simulink model "LunarLanderLQRKalman"  (R2022b)
settings: Solver=ode45  StartTime=0.0  StopTime=50  RelTol=1e-2
undefined symbols (not defined in the file): A, B, C, Kp, L, L_tK
libraries: simulink x4
settings Model: Creator=marco  LastModifiedBy=marco

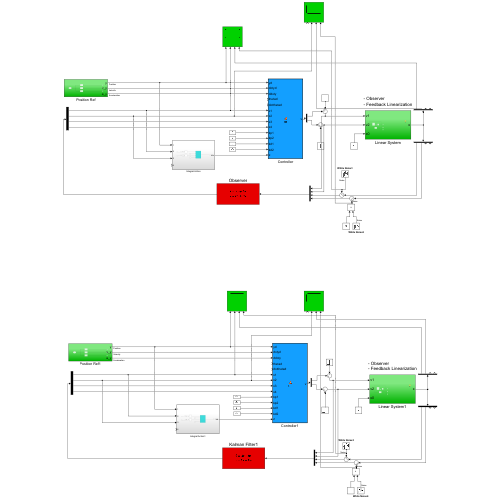
[thumbnail: Simulink's stored preview of the top-level diagram]
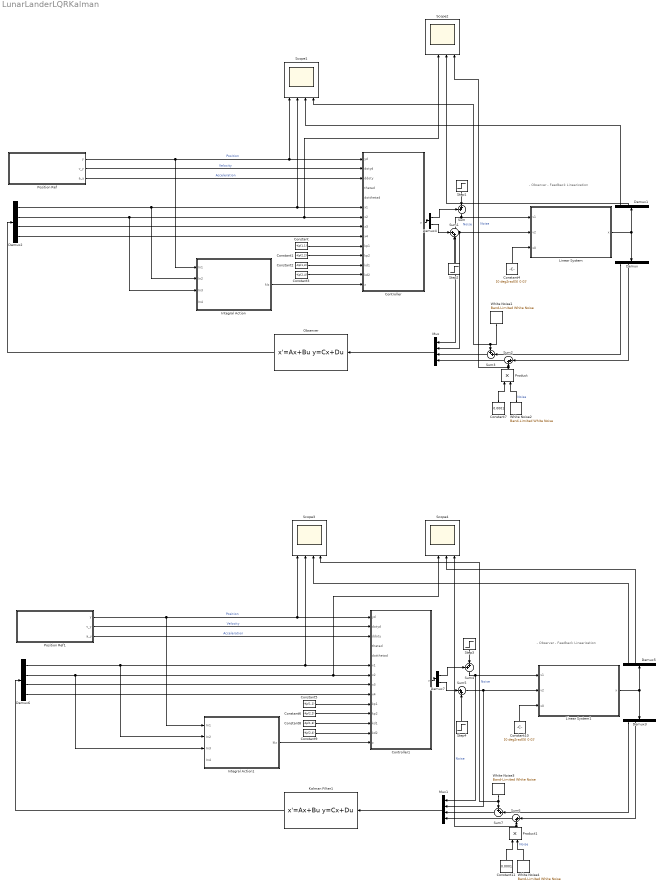
== system LunarLanderLQRKalman ==
  note: - Observer
      | - Feedback Linearization
  note: - Observer
      | - Feedback Linearization
  Constant : Constant  Value=-Kp(1,1)
  Constant1 : Constant  Value=-Kp(2,2)
  Constant10 : Constant  Value=[0 deg2rad(5) 0 0]'
  Constant11 : Constant  Value=0.0001
  Constant2 : Constant  Value=-Kp(1,3)
  Constant3 : Constant  Value=-Kp(2,4)
  Constant4 : Constant  Value=[0 deg2rad(5) 0 0]'
  Constant5 : Constant  Value=-Kp(1,1)
  Constant6 : Constant  Value=-Kp(2,2)
  Constant7 : Constant  Value=0.0001
  Constant8 : Constant  Value=-Kp(1,3)
  Constant9 : Constant  Value=-Kp(2,4)
  Controller : MATLAB Function  TreatAsAtomicUnit=on
  Controller1 : MATLAB Function  TreatAsAtomicUnit=on
  Demux{,1..3,5..6} (6 alike) : Demux
  Demux4 : Demux  Outputs=2
  Demux7 : Demux  Outputs=2
  Integral Action : Subsystem
  Integral Action1 : Subsystem
  Kalman Filter1 : StateSpace  A=A-L_tK*C  B=[B L_tK]  C=eye(4)  D=zeros(4)  InitialCondition=0
  Linear System : Subsystem
  Linear System1 : Subsystem
  Mux : Mux
  Mux1 : Mux
  Observer : StateSpace  A=A-L*C  B=[B L]  C=eye(4)  D=zeros(4)  InitialCondition=0
  Position Ref : Subsystem
  Position Ref1 : Subsystem
  Product : Product
  Product1 : Product
  Scope{1..4} (4 alike) : Scope  NumInputPorts=4
  Step1 : Step  After=10  SampleTime=0
  Step2 : Step  After=deg2rad(1)  SampleTime=0
  Step3 : Step  After=10  SampleTime=0
  Step4 : Step  After=deg2rad(1)  SampleTime=0
  Sum{,3..4,7} (4 alike) : Sum  Inputs=++|
  Sum{1..2,5..6} (4 alike) : Sum  Inputs=|++
  White Noise{1..4} (4 alike) : simulink/Sources/Band-Limited White Noise  Cov=[2]  Ts=0.1  seed=[213132]
  wires:
  Constant7/1 -> Product/1
  White Noise2/1 -> Product/2  "Noise"
  Position Ref/1(y) -> Controller/1(yd), Scope1/1, Integral Action/1(In1)  "Position"
  Demux4/1 -> Sum/1
  Demux1/2 -> Scope2/3
  Mux/1 -> Observer/1
  Sum1/1 -> Linear System/2(v2), Mux/2
  Integral Action/1(kIz) -> Controller/14(z)
  Controller/1(v) -> Demux4/1
  Demux2/4 -> Controller/9(x4)
  Constant1/1 -> Controller/11(kp2)
  Constant2/1 -> Controller/12(kd1)
  Constant4/1 -> Linear System/3(x0)
  Position Ref/3(a_y) -> Controller/3(ddoty)  "Acceleration"
  Observer/1 -> Demux2/1
  Position Ref/2(v_y) -> Controller/2(dotyd)  "Velocity"
  Demux2/3 -> Controller/8(x3)
  Constant3/1 -> Controller/13(kd2)
  Linear System/1(x) -> Demux/1, Demux1/1
  Demux/1 -> Sum3/2
  Demux1/1 -> Scope1/3
  Step1/1 -> Sum/2
  Constant/1 -> Controller/10(kp1)
  Demux4/2 -> Sum1/1
  Demux2/2 -> Controller/7(x2), Scope2/2, Integral Action/3(In3)
  Sum/1 -> Linear System/1(v1), Mux/1
  Demux2/1 -> Scope1/2, Controller/6(x1), Integral Action/2(In2)
  Step2/1 -> Sum1/2
  Demux/2 -> Sum2/1
  Sum2/1 -> Mux/4
  Product/1 -> Scope2/4, Sum2/2  "Noise"
  Sum3/1 -> Mux/3
  White Noise1/1 -> Scope1/4, Sum3/1  "Noise"
  Constant8/1 -> Controller1/12(kd1)
  Integral Action1/1(kIz) -> Controller1/14(z)
  Controller1/1(v) -> Demux7/1
  Sum5/1 -> Mux1/2, Linear System1/2(v2)
  Constant5/1 -> Controller1/10(kp1)
  Demux7/2 -> Sum5/1
  Sum4/1 -> Mux1/1, Linear System1/1(v1)
  Demux6/2 -> Scope4/2, Controller1/7(x2), Integral Action1/3(In3)
  Constant9/1 -> Controller1/13(kd2)
  Position Ref1/2(v_y) -> Controller1/2(dotyd)  "Velocity"
  Kalman Filter1/1 -> Demux6/1
  Step3/1 -> Sum4/2
  Linear System1/1(x) -> Demux3/1, Demux5/1
  Position Ref1/3(a_y) -> Controller1/3(ddoty)  "Acceleration"
  Demux6/3 -> Controller1/8(x3)
  Position Ref1/1(y) -> Controller1/1(yd), Scope3/1, Integral Action1/1(In1)  "Position"
  Sum7/1 -> Mux1/3
  Demux6/4 -> Controller1/9(x4)
  Demux3/2 -> Sum6/1
  Demux5/2 -> Scope4/3
  Step4/1 -> Sum5/2
  Demux7/1 -> Sum4/1
  Demux6/1 -> Scope3/2, Controller1/6(x1), Integral Action1/2(In2)
  Mux1/1 -> Kalman Filter1/1
  Demux3/1 -> Sum7/2
  White Noise4/1 -> Product1/2  "Noise"
  Constant11/1 -> Product1/1
  Sum6/1 -> Mux1/4
  Constant10/1 -> Linear System1/3(x0)
  Product1/1 -> Scope4/4, Sum6/2  "Noise"
  White Noise3/1 -> Scope3/4, Sum7/1  "Noise"
  Constant6/1 -> Controller1/11(kp2)
  Demux5/1 -> Scope3/3

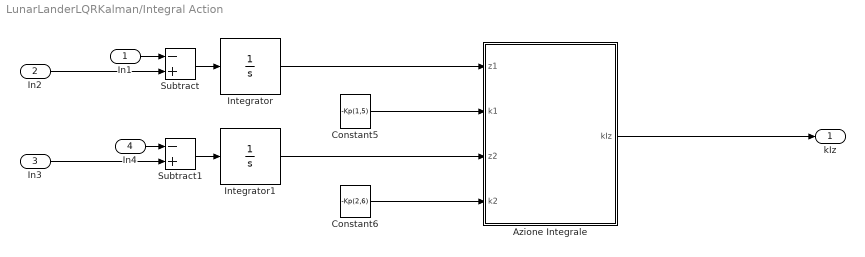
== system LunarLanderLQRKalman/Integral Action ==
  In1 : Inport
  In2 : Inport  Port=2
  In3 : Inport  Port=3
  In4 : Inport  Port=4
  Azione Integrale : MATLAB Function  TreatAsAtomicUnit=on
  Constant5 : Constant  Value=-Kp(1,5)
  Constant6 : Constant  Value=-Kp(2,6)
  Integrator : Integrator
  Integrator1 : Integrator
  Subtract : Sum  Inputs=-+
  Subtract1 : Sum  Inputs=-+
  kIz : Outport
  wires:
  Integrator/1 -> Azione Integrale/1(z1)
  Constant6/1 -> Azione Integrale/4(k2)
  Integrator1/1 -> Azione Integrale/3(z2)
  Subtract1/1 -> Integrator1/1
  Constant5/1 -> Azione Integrale/2(k1)
  Subtract/1 -> Integrator/1
  In3/1 -> Subtract1/2
  In4/1 -> Subtract1/1
  In1/1 -> Subtract/1
  Azione Integrale/1(kIz) -> kIz/1
  In2/1 -> Subtract/2

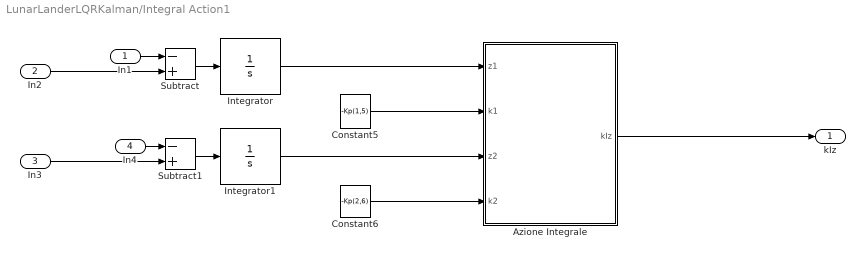
== system LunarLanderLQRKalman/Integral Action1 ==
  In1 : Inport
  In2 : Inport  Port=2
  In3 : Inport  Port=3
  In4 : Inport  Port=4
  Azione Integrale : MATLAB Function  TreatAsAtomicUnit=on
  Constant5 : Constant  Value=-Kp(1,5)
  Constant6 : Constant  Value=-Kp(2,6)
  Integrator : Integrator
  Integrator1 : Integrator
  Subtract : Sum  Inputs=-+
  Subtract1 : Sum  Inputs=-+
  kIz : Outport
  wires:
  Integrator/1 -> Azione Integrale/1(z1)
  Constant6/1 -> Azione Integrale/4(k2)
  Integrator1/1 -> Azione Integrale/3(z2)
  Subtract1/1 -> Integrator1/1
  Constant5/1 -> Azione Integrale/2(k1)
  Subtract/1 -> Integrator/1
  In3/1 -> Subtract1/2
  In4/1 -> Subtract1/1
  In1/1 -> Subtract/1
  Azione Integrale/1(kIz) -> kIz/1
  In2/1 -> Subtract/2

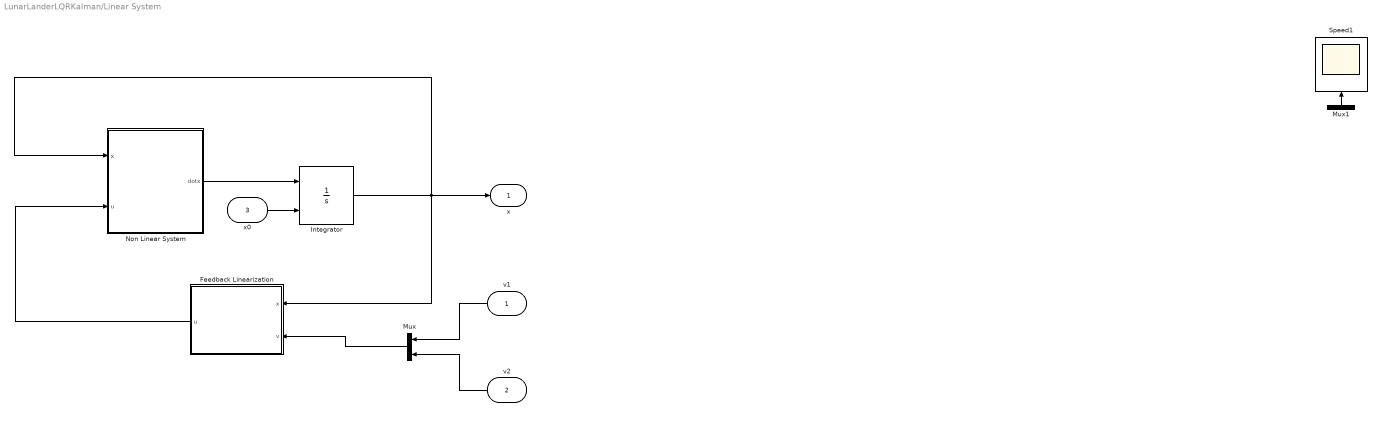
== system LunarLanderLQRKalman/Linear System ==
  v1 : Inport
  v2 : Inport  Port=2
  x0 : Inport  Port=3
  Feedback Linearization : MATLAB Function  TreatAsAtomicUnit=on
  Integrator : Integrator  InitialConditionSource=external  InitialCondition=[0 0 0 0]'
  Mux : Mux  Inputs=2
  Mux1 : Mux  Inputs=2
  Non Linear System : MATLAB Function  TreatAsAtomicUnit=on
  Speed1 : Scope
  x : Outport
  wires:
  Feedback Linearization/1(u) -> Non Linear System/2(u)
  Integrator/1 -> Non Linear System/1(x), x/1, Feedback Linearization/1(x)
  Non Linear System/1(dotx) -> Integrator/1
  x0/1 -> Integrator/2
  v1/1 -> Mux/1
  v2/1 -> Mux/2
  Mux/1 -> Feedback Linearization/2(v)
  Mux1/1 -> Speed1/1

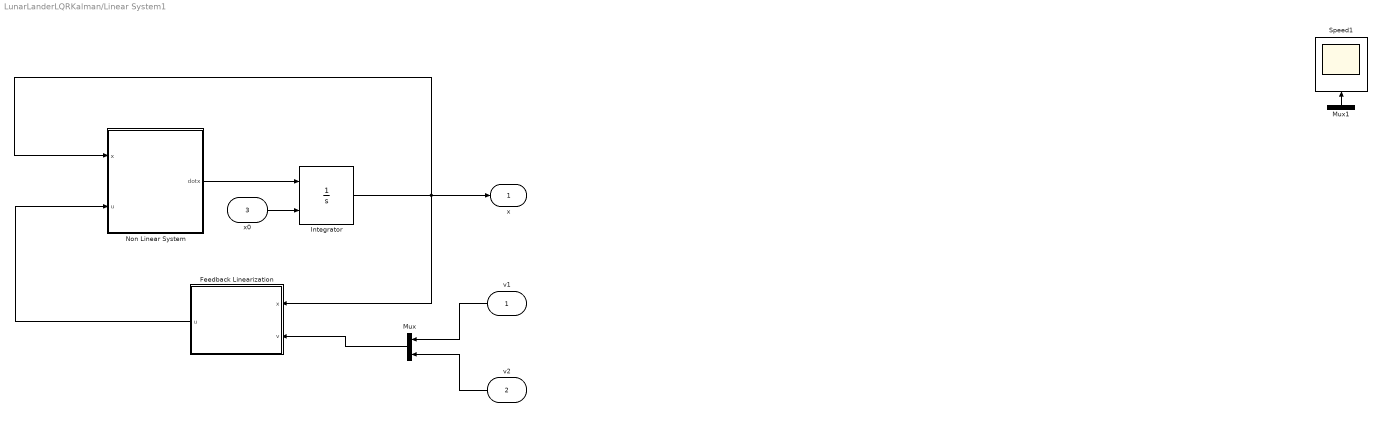
== system LunarLanderLQRKalman/Linear System1 ==
  v1 : Inport
  v2 : Inport  Port=2
  x0 : Inport  Port=3
  Feedback Linearization : MATLAB Function  TreatAsAtomicUnit=on
  Integrator : Integrator  InitialConditionSource=external  InitialCondition=[0 0 0 0]'
  Mux : Mux  Inputs=2
  Mux1 : Mux  Inputs=2
  Non Linear System : MATLAB Function  TreatAsAtomicUnit=on
  Speed1 : Scope
  x : Outport
  wires:
  Feedback Linearization/1(u) -> Non Linear System/2(u)
  Integrator/1 -> Non Linear System/1(x), x/1, Feedback Linearization/1(x)
  Non Linear System/1(dotx) -> Integrator/1
  x0/1 -> Integrator/2
  v1/1 -> Mux/1
  v2/1 -> Mux/2
  Mux/1 -> Feedback Linearization/2(v)
  Mux1/1 -> Speed1/1

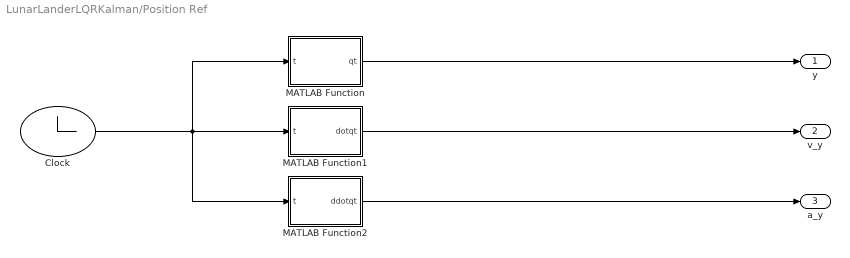
== system LunarLanderLQRKalman/Position Ref ==
  Clock : Clock
  MATLAB Function : MATLAB Function  TreatAsAtomicUnit=on
  MATLAB Function1 : MATLAB Function  TreatAsAtomicUnit=on
  MATLAB Function2 : MATLAB Function  TreatAsAtomicUnit=on
  y : Outport
  v_y : Outport  Port=2
  a_y : Outport  Port=3
  wires:
  MATLAB Function/1(qt) -> y/1
  MATLAB Function1/1(dotqt) -> v_y/1
  MATLAB Function2/1(ddotqt) -> a_y/1
  Clock/1 -> MATLAB Function2/1(t), MATLAB Function1/1(t), MATLAB Function/1(t)

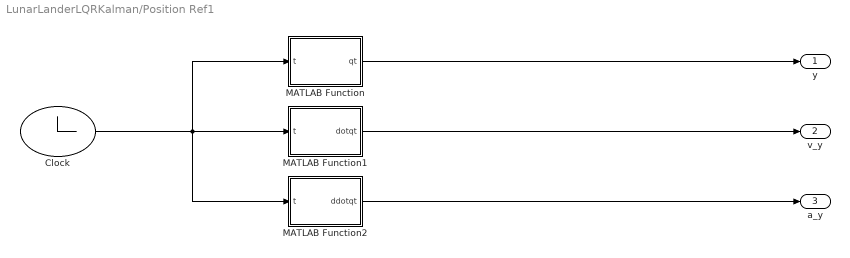
== system LunarLanderLQRKalman/Position Ref1 ==
  Clock : Clock
  MATLAB Function : MATLAB Function  TreatAsAtomicUnit=on
  MATLAB Function1 : MATLAB Function  TreatAsAtomicUnit=on
  MATLAB Function2 : MATLAB Function  TreatAsAtomicUnit=on
  y : Outport
  v_y : Outport  Port=2
  a_y : Outport  Port=3
  wires:
  MATLAB Function/1(qt) -> y/1
  MATLAB Function1/1(dotqt) -> v_y/1
  MATLAB Function2/1(ddotqt) -> a_y/1
  Clock/1 -> MATLAB Function2/1(t), MATLAB Function1/1(t), MATLAB Function/1(t)

== matlab function LunarLanderLQRKalman/Linear System1/Non Linear System ==
  data: x input; u input; dotx output
function dotx  = fcn(x, u)

g = 1.62;
m = 23000;
J = 100000;
c = 1000;

y = x(1)
theta = x(2)
v = x(3)
w = x(4)

doty = v
dottheta = w
dotv = (u(1)*sin(theta)+u(2)*cos(theta)-m*g-c*v)/m
dotw = 4*u(1)/J

dotx = [doty, dottheta, dotv, dotw]';

== matlab function LunarLanderLQRKalman/Position Ref/MATLAB Function ==
  data: t input; qt output
function qt = fcn(t)

tf = 20 %s
dotqc = 8 %m/s
qi = 0 %m - valore integratore per y_0
qf = 100 %m

tc = tf - (qf - qi)/dotqc

ddotqc = dotqc/tc

q1 = qi + 0.5 * ddotqc * t^2;
q2 = qi + ddotqc*tc*(t-tc/2);
q3 = qi + ddotqc*tc*(tf-tc-tc/2) + dotqc*(t-(tf-tc))-0.5*ddotqc*(t-(tf-tc))^2;

if t>=0 && t<=tc
    qt = q1
elseif t>tc && t<=(tf-tc)
    qt = q2
elseif t>(tf-tc) && t<=tf
    qt = q3
elseif t>tf
    qt = 100
else 
    qt = 0
end

== matlab function LunarLanderLQRKalman/Position Ref/MATLAB Function1 ==
  data: t input; dotqt output
function dotqt = fcn(t)

tf = 20 %s
dotqc = 8 %m/s
qi = 0 %m - valore integratore per y_0
qf = 100 %m

tc = tf - (qf - qi)/dotqc

ddotqc = dotqc/tc

dotq1 = ddotqc*t;
dotq2 = dotqc;
dotq3 = dotqc-ddotqc*(t-(tf-tc));

if t>=0 && t<=tc
    dotqt = dotq1
elseif t>tc && t<=(tf-tc)
    dotqt = dotq2
elseif t>(tf-tc) && t<=tf
    dotqt = dotq3
else 
    dotqt = 0
end

== matlab function LunarLanderLQRKalman/Position Ref/MATLAB Function2 ==
  data: t input; ddotqt output
function ddotqt = fcn(t)

tf = 20 %s
dotqc = 8 %m/s
qi = 0 %m - valore integratore per y_0
qf = 100 %m

tc = tf - (qf - qi)/dotqc

ddotqc = dotqc/tc

ddotq1 = ddotqc;
ddotq2 = 0;
ddotq3 = -ddotqc;

if t>=0 && t<=tc
    ddotqt = ddotq1
elseif t>tc && t<=(tf-tc)
    ddotqt = ddotq2
elseif t>(tf-tc) && t<=tf
    ddotqt = ddotq3
else 
    ddotqt = 0
end

== matlab function LunarLanderLQRKalman/Position Ref1/MATLAB Function ==
  data: t input; qt output
function qt = fcn(t)

tf = 20 %s
dotqc = 8 %m/s
qi = 0 %m - valore integratore per y_0
qf = 100 %m

tc = tf - (qf - qi)/dotqc

ddotqc = dotqc/tc

q1 = qi + 0.5 * ddotqc * t^2;
q2 = qi + ddotqc*tc*(t-tc/2);
q3 = qi + ddotqc*tc*(tf-tc-tc/2) + dotqc*(t-(tf-tc))-0.5*ddotqc*(t-(tf-tc))^2;

if t>=0 && t<=tc
    qt = q1
elseif t>tc && t<=(tf-tc)
    qt = q2
elseif t>(tf-tc) && t<=tf
    qt = q3
elseif t>tf
    qt = 100
else 
    qt = 0
end

== matlab function LunarLanderLQRKalman/Position Ref1/MATLAB Function1 ==
  data: t input; dotqt output
function dotqt = fcn(t)

tf = 20 %s
dotqc = 8 %m/s
qi = 0 %m - valore integratore per y_0
qf = 100 %m

tc = tf - (qf - qi)/dotqc

ddotqc = dotqc/tc

dotq1 = ddotqc*t;
dotq2 = dotqc;
dotq3 = dotqc-ddotqc*(t-(tf-tc));

if t>=0 && t<=tc
    dotqt = dotq1
elseif t>tc && t<=(tf-tc)
    dotqt = dotq2
elseif t>(tf-tc) && t<=tf
    dotqt = dotq3
else 
    dotqt = 0
end

== matlab function LunarLanderLQRKalman/Position Ref1/MATLAB Function2 ==
  data: t input; ddotqt output
function ddotqt = fcn(t)

tf = 20 %s
dotqc = 8 %m/s
qi = 0 %m - valore integratore per y_0
qf = 100 %m

tc = tf - (qf - qi)/dotqc

ddotqc = dotqc/tc

ddotq1 = ddotqc;
ddotq2 = 0;
ddotq3 = -ddotqc;

if t>=0 && t<=tc
    ddotqt = ddotq1
elseif t>tc && t<=(tf-tc)
    ddotqt = ddotq2
elseif t>(tf-tc) && t<=tf
    ddotqt = ddotq3
else 
    ddotqt = 0
end

== matlab function LunarLanderLQRKalman/Linear System/Feedback Linearization ==
  data: x input; v input; u output
function u = fcn(x, v)

g = 1.62;
m = 23000;
J = 100000;
c = 1000;

Q = [sin(x(2))/m cos(x(2))/m;4/J 0]
Qinv = Q^-1

A = [-(g-c*x(3)/m); 0]
ueq = Qinv*(-A+v)

u = [ueq(1); ueq(2)];

== matlab function LunarLanderLQRKalman/Linear System/Non Linear System ==
  data: x input; u input; dotx output
function dotx  = fcn(x, u)

g = 1.62;
m = 23000;
J = 100000;
c = 1000;

y = x(1)
theta = x(2)
v = x(3)
w = x(4)

doty = v
dottheta = w
dotv = (u(1)*sin(theta)+u(2)*cos(theta)-m*g-c*v)/m
dotw = 4*u(1)/J

dotx = [doty, dottheta, dotv, dotw]';

== matlab function LunarLanderLQRKalman/Controller ==
  data: yd input; dotyd input; ddoty input; thetad input; dotthetad input; x1 input; x2 input; x3 input; x4 input; v output; kp1 input; kp2 input; kd1 input; kd2 input; z input
function v = fcn(yd, dotyd, ddoty, thetad, dotthetad, x1, x2, x3, x4, kp1, kp2, kd1, kd2, z)

v1 = kp1*(x1-yd) + kd1*(x3-dotyd) + ddoty + z(1)
v2 = kp2*(x2-thetad) + kd2*(x4-dotthetad) + z(2)

v = [v1; v2]

== matlab function LunarLanderLQRKalman/Integral Action/Azione Integrale ==
  data: z1 input; kIz output; k1 input; z2 input; k2 input
function kIz = fcn(z1, k1, z2, k2)

kIz = [z1*k1; z2*k2];

== matlab function LunarLanderLQRKalman/Controller1 ==
  data: yd input; dotyd input; ddoty input; thetad input; dotthetad input; x1 input; x2 input; x3 input; x4 input; v output; kp1 input; kp2 input; kd1 input; kd2 input; z input
function v = fcn(yd, dotyd, ddoty, thetad, dotthetad, x1, x2, x3, x4, kp1, kp2, kd1, kd2, z)

v1 = kp1*(x1-yd) + kd1*(x3-dotyd) + ddoty + z(1)
v2 = kp2*(x2-thetad) + kd2*(x4-dotthetad) + z(2)

v = [v1; v2]

== matlab function LunarLanderLQRKalman/Integral Action1/Azione Integrale ==
  data: z1 input; kIz output; k1 input; z2 input; k2 input
function kIz = fcn(z1, k1, z2, k2)

kIz = [z1*k1; z2*k2];

== matlab function LunarLanderLQRKalman/Linear System1/Feedback Linearization ==
  data: x input; v input; u output
function u = fcn(x, v)

g = 1.62;
m = 23000;
J = 100000;
c = 1000;

Q = [sin(x(2))/m cos(x(2))/m;4/J 0]
Qinv = Q^-1

A = [-(g-c*x(3)/m); 0]
ueq = Qinv*(-A+v)

u = [ueq(1); ueq(2)];
